simulink model "Ind_prob01In3op4"  (R2019a)
settings: Solver=FixedStepDiscrete  StartTime=0.0  StopTime=10.0  FixedStep=1  RelTol=1e-3
undefined symbols (not defined in the file): Compareto3, Compareto4, Compareto8, in3op4, in4op8, in8op16, notequalto0
settings Model: DataDictionary=IP_1ip3op4.sldd  Creator=Hp  LastModifiedBy=Hp
settings DataIOCC: SaveFormat=Array  SaveOutput=off
settings OptimizationCC: DefaultParameterBehavior=Inlined  EnhancedBackFolding=on  PassReuseOutputArgsAs=Individual arguments  OptimizeBlockOrder=speed  DifferentSizesBufferReuse=on  OptimizationCustomize=off
settings DebuggingCC: ParameterTunabilityLossMsg=error
settings SFSimCC: MATLABDynamicMemAlloc=off
settings RTWCC: SystemTargetFile=ert.tlc  GenCodeOnly=on  PackageGeneratedCodeAndArtifacts=on  TemplateMakefile=ert_default_tmf  GenerateReport=on  IncludeHyperlinkInReport=on  LaunchReport=on  GenerateTraceInfo=on  GenerateTraceReport=on  GenerateTraceReportSl=on  GenerateTraceReportSf=on  GenerateTraceReportEml=on
settings CodeAppCC: ForceParamTrailComments=on  IgnoreCustomStorageClasses=off  OperatorAnnotations=on  SimulinkDataObjDesc=on  SFDataObjDesc=on  InsertBlockDesc=on
settings ERTTargetCC: TargetLangStandard=C99 (ISO)  GenerateSampleERTMain=on  InlinedParameterPlacement=NonHierarchical  ERTCustomFileTemplate=example_file_process.tlc
settings ConfigComp: CovEnable=on  RecordCoverage=on  CovMetricSettings=dcmw  CovHtmlReporting=on  CovCumulativeReport=on  CovModelRefEnable=on

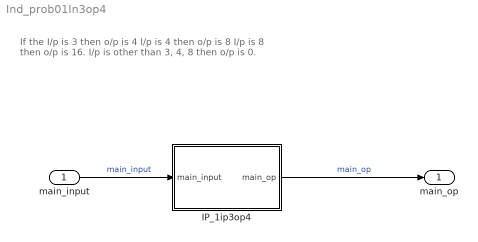
== system Ind_prob01In3op4 ==
  note: If the I/p is 3 then o/p is 4
      | I/p is 4 then o/p is 8
      | I/p is 8 then o/p is 16.
      | I/p is other than 3, 4, 8 then o/p is 0.
  main_input : Inport
  IP_1ip3op4 : Subsystem  TreatAsAtomicUnit=on
  main_op : Outport
  wires:
  main_input/1 -> IP_1ip3op4/1(main_input)  "main_input"
  IP_1ip3op4/1(main_op) -> main_op/1  "main_op"

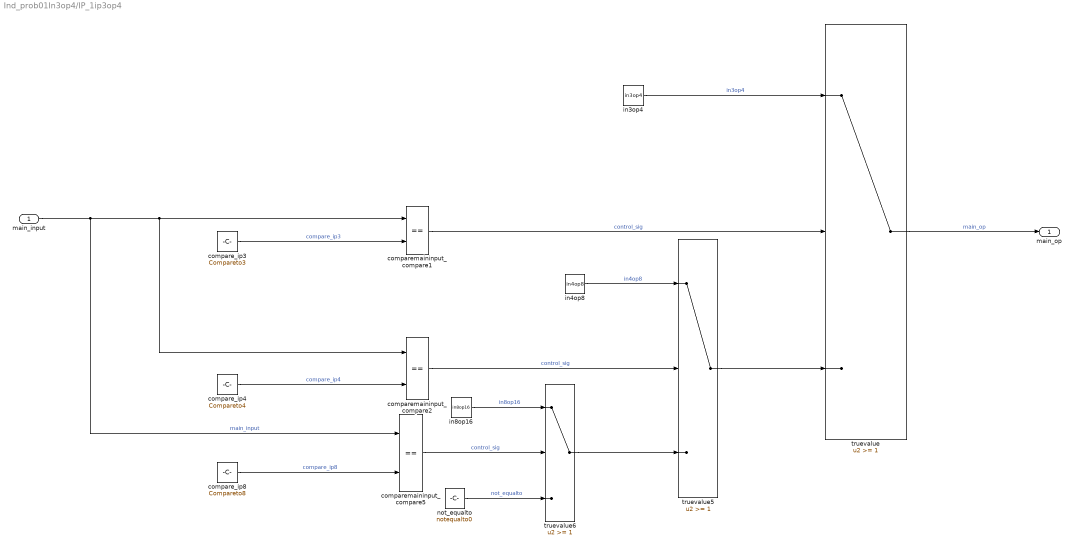
== system Ind_prob01In3op4/IP_1ip3op4 ==
  main_input : Inport
  compare_ip3 : Constant  Value=Compareto3
  compare_ip4 : Constant  Value=Compareto4
  compare_ip8 : Constant  Value=Compareto8
  comparemaininput_compare1 : RelationalOperator  Operator===  OutDataTypeStr=boolean  RndMeth=Simplest
  comparemaininput_compare2 : RelationalOperator  Operator===  OutDataTypeStr=boolean  RndMeth=Simplest
  comparemaininput_compare5 : RelationalOperator  Operator===  OutDataTypeStr=boolean  RndMeth=Simplest
  in3op4 : Constant  Value=in3op4
  in4op8 : Constant  Value=in4op8
  in8op16 : Constant  Value=in8op16
  not_equalto : Constant  Value=notequalto0
  truevalue : Switch  Threshold=1
  truevalue5 : Switch  Threshold=1
  truevalue6 : Switch  Threshold=1
  main_op : Outport
  wires:
  main_input/1 -> comparemaininput_compare1/1, comparemaininput_compare2/1, comparemaininput_compare5/1  "main_input"
  comparemaininput_compare2/1 -> truevalue5/2  "control_sig"
  in3op4/1 -> truevalue/1  "in3op4"
  compare_ip8/1 -> comparemaininput_compare5/2  "compare_ip8"
  truevalue6/1 -> truevalue5/3
  compare_ip4/1 -> comparemaininput_compare2/2  "compare_ip4"
  truevalue5/1 -> truevalue/3
  comparemaininput_compare5/1 -> truevalue6/2  "control_sig"
  in4op8/1 -> truevalue5/1  "in4op8"
  compare_ip3/1 -> comparemaininput_compare1/2  "compare_ip3"
  in8op16/1 -> truevalue6/1  "in8op16"
  truevalue/1 -> main_op/1  "main_op"
  not_equalto/1 -> truevalue6/3  "not_equalto"
  comparemaininput_compare1/1 -> truevalue/2  "control_sig"
